simulink model "feedback_linearization"  (R2023b)
settings: Solver=FixedStepAuto  StartTime=0.0  StopTime=15  FixedStep=0.001  RelTol=1e-3
values from neighbouring files (symbols this model uses):
  a = [q1, q2, q3, J]    [observer_for_disturbance_par.m]    (also in openloop_control_par.m; state_feedback_around_eq_par.m)
  x0 = [2; 200; 0]    [observer_for_disturbance_par.m]    (also in openloop_control_par.m = [ 2 ; 200 ]; state_feedback_around_eq_par.m = [2; 200])
settings Model: Creator=peterparker  LastModifiedBy=peterparker

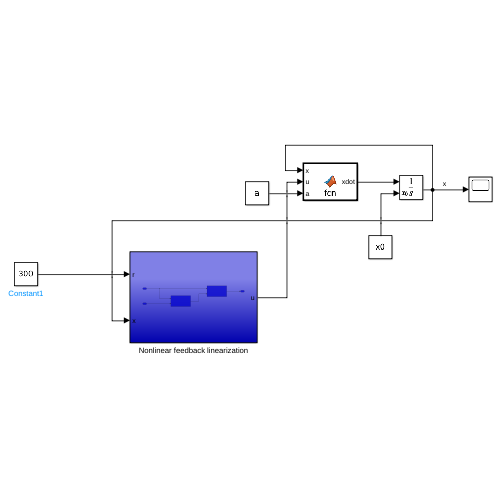
[thumbnail: Simulink's stored preview of the top-level diagram]
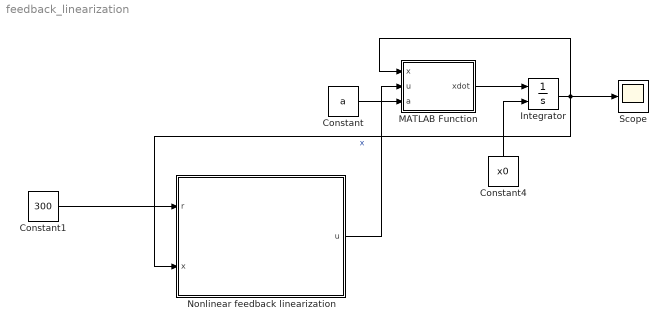
== system feedback_linearization ==
  Constant : Constant  Value=a
  Constant1 : Constant  Value=300
  Constant4 : Constant  Value=x0
  Integrator : Integrator  InitialConditionSource=external
  MATLAB Function : MATLAB Function  TreatAsAtomicUnit=on
  Nonlinear feedback linearization : Subsystem
  Scope : Scope
  wires:
  MATLAB Function/1(xdot) -> Integrator/1
  Constant4/1 -> Integrator/2
  Integrator/1 -> Nonlinear feedback linearization/2(x), Scope/1, MATLAB Function/1(x)  "x"
  Constant/1 -> MATLAB Function/3(a)
  Nonlinear feedback linearization/1(u) -> MATLAB Function/2(u)
  Constant1/1 -> Nonlinear feedback linearization/1(r)

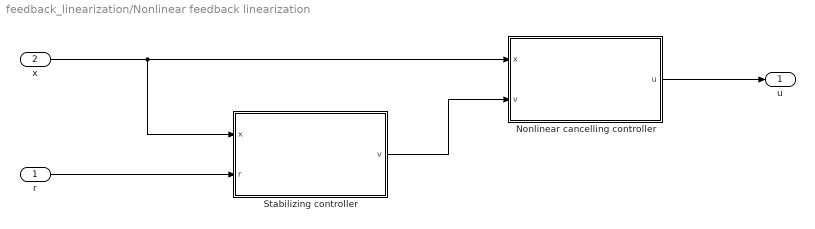
== system feedback_linearization/Nonlinear feedback linearization ==
  r : Inport
  x : Inport  Port=2
  Nonlinear cancelling controller : Subsystem
  Stabilizing controller : Subsystem
  u : Outport
  wires:
  Nonlinear cancelling controller/1(u) -> u/1
  x/1 -> Stabilizing controller/1(x), Nonlinear cancelling controller/1(x)
  Stabilizing controller/1(v) -> Nonlinear cancelling controller/2(v)
  r/1 -> Stabilizing controller/2(r)

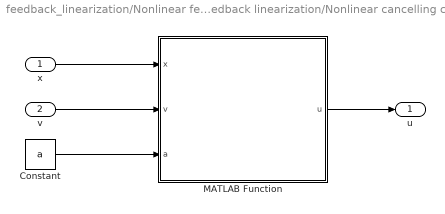
== system feedback_linearization/Nonlinear feedback linearization/Nonlinear cancelling controller ==
  x : Inport
  v : Inport  Port=2
  Constant : Constant  Value=a  VectorParams1D=off
  MATLAB Function : MATLAB Function  TreatAsAtomicUnit=on
  u : Outport
  wires:
  x/1 -> MATLAB Function/1(x)
  v/1 -> MATLAB Function/2(v)
  MATLAB Function/1(u) -> u/1
  Constant/1 -> MATLAB Function/3(a)

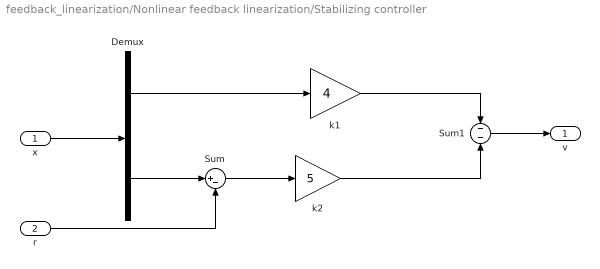
== system feedback_linearization/Nonlinear feedback linearization/Stabilizing controller ==
  x : Inport
  r : Inport  Port=2
  Demux : Demux  Outputs=2
  Sum : Sum  Inputs=|+-
  Sum1 : Sum  Inputs=--
  k1 : Gain  Gain=4
  k2 : Gain  Gain=5
  v : Outport
  wires:
  x/1 -> Demux/1
  Sum1/1 -> v/1
  k1/1 -> Sum1/1
  k2/1 -> Sum1/2
  Sum/1 -> k2/1
  Demux/1 -> k1/1
  Demux/2 -> Sum/1
  r/1 -> Sum/2

== matlab function feedback_linearization/Nonlinear feedback linearization/Nonlinear cancelling controller/MATLAB Function ==
  data: x input; v input; u output; a input
function u = c_lin(x,v,a)

% a is the vector of constant parameters
q1 = a(1);

% cancelling controller
u = q1*x(1)*x(2) + v;

== matlab function feedback_linearization/MATLAB Function ==
  data: x input; u input; xdot output; a input
function xdot = fcn(x,u, a)

q1 = a(1);
q2 = a(2);
q3 = a(3);
J = a(4);


xdot = [-q1 * x(2) * x(1) + u; 
        q2/J * x(1) - q3/J * x(2)];
